simulink model "UDP_Client_Send2"  (R2015a)
settings: Solver=FixedStepDiscrete  SolverMode=SingleTasking  StartTime=0.0  StopTime=10.0  FixedStep=1e-3  RelTol=1e-3
libraries: mbed_ethernet_udp x3, simulink x1, mbed_lib x1, mbed_targets_stm_arch_max x1
settings Model: Creator=oh  LastModifiedBy=oh
settings OptimizationCC: OptimizeModelRefInitCode=on  LifeSpan=1
settings HardwareCC: ProdLargestAtomicInteger=Long  ProdLargestAtomicFloat=Double  ProdEndianess=LittleEndian  ProdHWDeviceType=ARM Compatible->ARM Cortex
settings RTWCC: SystemTargetFile=mbed.tlc  TemplateMakefile=mbed.tmf  Description=Mbed Target (Embedded Target)  TargetLang=C++
settings CodeAppCC: IgnoreCustomStorageClasses=off
settings STFCustomTargetCC: CombineOutputUpdateFcns=on  SupportContinuousTime=off  SupportVariableSizeSignals=off  SystemTargetFile=mbed.tlc
settings ERTTargetCC: SupportContinuousTime=off  SupportVariableSizeSignals=off  ERTCustomFileTemplate=mbed_file_process.tlc

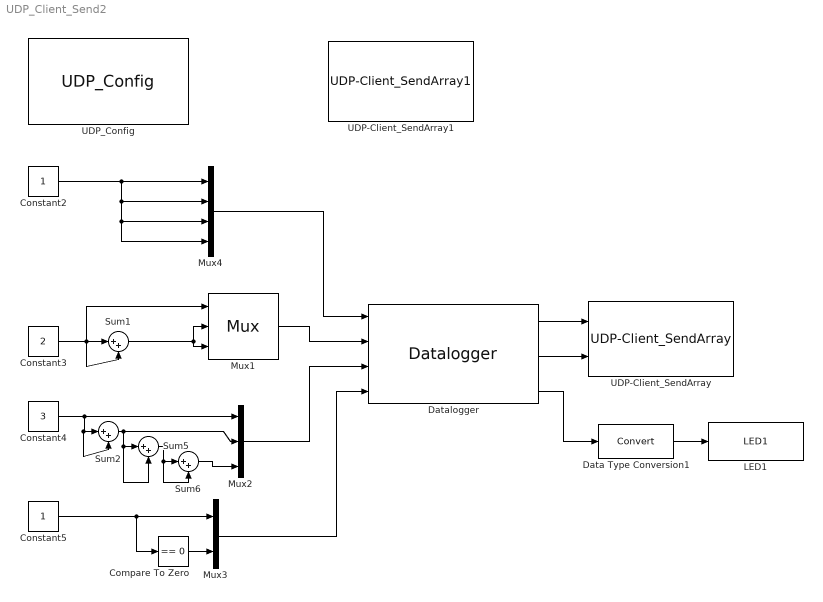
== system UDP_Client_Send2 ==
  Compare To Zero : simulink/Logic and Bit Operations/Compare To Zero  relop===  OutDataTypeStr=boolean
  Constant2 : Constant  OutDataTypeStr=uint8
  Constant3 : Constant  Value=2  OutDataTypeStr=int16
  Constant4 : Constant  Value=3
  Constant5 : Constant  OutDataTypeStr=boolean
  Data Type Conversion1 : DataTypeConversion
  Datalogger : mbed_lib/Utilities/Datalogger  TypeInputPorts={ 'uint8' 4 'int16' 3 'double' 3 'bool' 2 }  TypeOfInputs={'4*uint8' '3*int16' '3*double' '2*bool'}  BufferSize=120  errEn=on  SampleTime=1
  LED1 : mbed_targets_stm_arch_max/LED1  Parameter1=0
  Mux1 : Mux  Inputs=3
      settings: DisplayOption=signals
  Mux2 : Mux  Inputs=3
  Mux3 : Mux  Inputs=2
  Mux4 : Mux
  Sum{1..2,5..6} (4 alike) : Sum  Inputs=|++
  UDP-Client_SendArray : mbed_ethernet_udp/UDP-Client_SendArray  sock_ID=2  numData=on  SampleTime=-1
  UDP-Client_SendArray1 : mbed_ethernet_udp/UDP-Client_SendArray1  des_IP='192.168.1.10'  des_port=7195  sock_ID=2
  UDP_Config : mbed_ethernet_udp/UDP_Config  Priority=0  sDHCP=on  DHCP=1  ip_addr='127.0.0.1'  sub_mask='255.255.255.0'  gateway='0.0.0.0'  DEFAULT_UDP_RECVMBOX_SIZE=8  TCPIP_THREAD_STACKSIZE=1024  TCPIP_THREAD_PRIO=Normal  PBUF_POOL_SIZE=5  TCP_MSS=1460
  wires:
  Sum1/1 -> Mux1/2, Mux1/3
  Sum2/1 -> Mux2/2, Sum5/2, Sum5/1
  Constant3/1 -> Sum1/2, Sum1/1, Mux1/1
  Constant4/1 -> Mux2/1, Sum2/2, Sum2/1
  Sum5/1 -> Sum6/2, Sum6/1
  Constant5/1 -> Compare To Zero/1, Mux3/1
  Sum6/1 -> Mux2/3
  Mux2/1 -> Datalogger/3
  Mux1/1 -> Datalogger/2
  Mux3/1 -> Datalogger/4
  Constant2/1 -> Mux4/4, Mux4/3, Mux4/2, Mux4/1
  Mux4/1 -> Datalogger/1
  Compare To Zero/1 -> Mux3/2
  Datalogger/1 -> UDP-Client_SendArray/1
  Datalogger/2 -> UDP-Client_SendArray/2
  Datalogger/3 -> Data Type Conversion1/1
  Data Type Conversion1/1 -> LED1/1
